simulink model "ssp_ad_scan"  (Simulink 6.5)
settings: Solver=VariableStepDiscrete  SolverMode=SingleTasking  StartTime=0.0  StopTime=10  RelTol=1e-3
undefined symbols (not defined in the file or in its folder): gcbh, xlBlockLoadCallback, xlGetSimulinkPeriod
libraries: xbsIndex_r4 x111, nort_sysgenlib x19
(part 1 of 2)
settings Model: Creator=nort  LastModifiedBy=nort
settings DebuggingCC: MultiTaskDSMMsg=warning  MultiTaskCondExecSysMsg=none
settings RTWCC: IncludeERTFirstTime=on

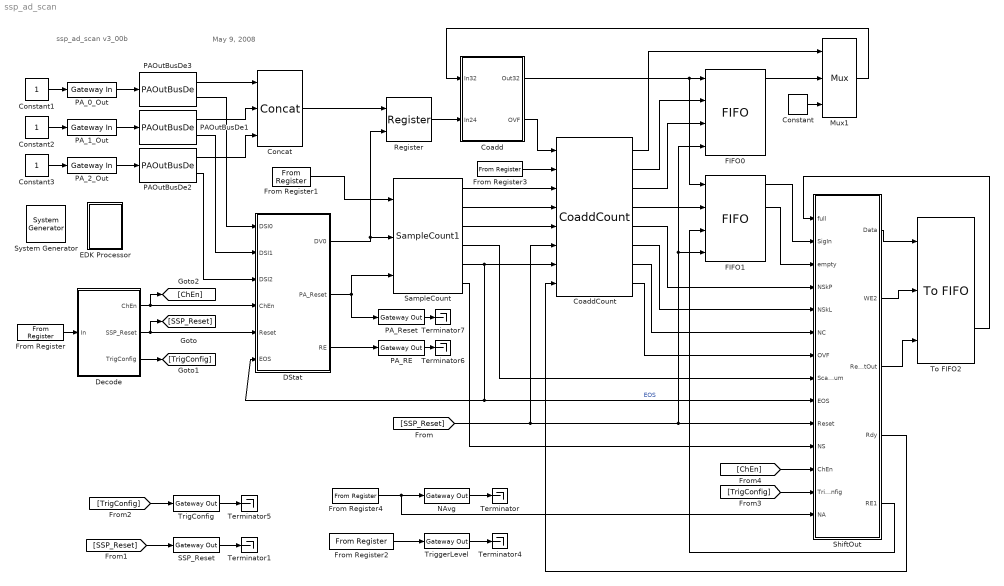
== system ssp_ad_scan ==
  note: May 9, 2008
  note: ssp_ad_scan v3_00b
  " System Generator" : xbsIndex_r4/ System Generator  Tag=genX  SystemSampleTime=-1  xilinxfamily=virtex4  part=xc4vlx25  speed=-10  package=ff668  synthesis_tool=XST  directory=./netlist  testbench=off  simulink_period=1  sysclk_period=10  incr_netlist=off  trim_vbits=Everywhere in SubSystem  dbl_ovrd=According to Block Masks  core_generation=According to Block Masks  run_coregen=off  deprecated_control=off  eval_field=0  block_type=sysgen
      settings: block_version=8.2
  Coadd : Subsystem
  CoaddCount : nort_sysgenlib/CoaddCount  SystemSampleTime=-1
  Concat : xbsIndex_r4/Concat  num_inputs=3  dbl_ovrd=off  block_type=concat
      settings: block_version=9.2.01
  Constant : xbsIndex_r4/Constant  arith_type=Unsigned  const=0  n_bits=96  bin_pt=0  explicit_period=off  period=1  equ=P=C  opselect=C  inp2=PCIN>>17  opr=+  inp1=P  carry=CIN  dbl_ovrd=off  block_type=constant
      settings: block_version=9.2.01
  Constant1 : Constant  Value=1  OutDataType=sfix(16)  ConRadixGroup=Use specified scaling  OutScaling=2^0  SampleTime=inf  FramePeriod=inf
  Constant2 : Constant  Value=1  OutDataType=sfix(16)  ConRadixGroup=Use specified scaling  OutScaling=2^0  SampleTime=inf  FramePeriod=inf
  Constant3 : Constant  Value=1  OutDataType=sfix(16)  ConRadixGroup=Use specified scaling  OutScaling=2^0  SampleTime=inf  FramePeriod=inf
  DStat : Subsystem
  Decode : Subsystem
  EDK Processor : Subsystem  LoadFcn=xlBlockLoadCallback(gcbh);  mask(Xilinx EDK Processor Block){xmp=, proc=, xbd=, mode=EDK pcore generation, MemVisToProc=<qt bgcolor="#FFFFFF"><div><img src="C:\Xilinx91i\dsptools\9.2.01.1028\sysgen\data\images\registerplus.gif"> &lt;&lt;Control&gt;&gt;<br></div><div><img src="C:\Xilinx91i\dsptools\9.2.01.1028\sysgen\data\images\registerminus.gif"> &lt;&lt;NAvg&gt;&gt;<br> <img src="C:\Xilinx91i\dsptools\9.2.01.1028\sysgen\data\images\parameters.gif"> Type : UFix_8_0<br></div><div><img src="C:\Xilinx91i\dsptools\9.2.01.1028\sysgen\data\images\registerplus.gif"> &lt;&lt;NetSamples&gt;&gt;<br></div><div><img src="C:\Xilinx91i\dsptools\9.2.01.1028\sysgen\data\images\registerplus.gif"> &lt;&lt;TriggerLevel&gt;&gt;<br></div><div><img src="C:\Xilinx91i\dsptools\9.2.01.1028\sysgen\data\images\registerplus.gif"> &lt;&lt;NCoadd&gt;&gt;<br></div><div><img src="C:\Xilinx91i\dsptools\9.2.01.1028\sysgen\data\images\fifoplus.gif"> &lt;&lt;SrcSignal&gt;&gt;<br></div></qt>, AvailableMemories=<empty>, launchGDB_sgadvanced=, launchGDB=off, cosim_mode_sgadvanced=, cosim_mode=Single Step, portInterfaceTable={'exposed'=>[],'portdir'=>[],'portname'=>[],'shortname'=>[]}, bus_type_sgadvanced=, bus_type=FSL, baseaddr=0x80000000, baseaddr_lock_sgadvanced=, baseaddr_lock=off, internalPortList={}, resetPolarity=0, memxtable={'mlist'=>['ssp_ad_scan/From Register','ssp_ad_scan/From Register4','ssp_ad_scan/From Register1','ssp_ad_scan/From Register2','ssp_ad_scan/From Register3','ssp_ad_scan/To FIFO2'],'mlname'=>['\'Control\'','\'NAvg\'','\'NetSamples\'','\'TriggerLevel\'','\'NCoadd\'','\'SrcSignal\''],'mlstate'=>[0.00000000000000000,1.0000000000000000,0.00000000000000000,0.00000000000000000,0.00000000000000000,0.00000000000000000]}, procinfo={'xmliface'=>'Xilinx//microblaze//iface.xml'}, fslifaceports=[0,0], memmapdirty=off, blockname=ssp_ad_scan_EDK_Processor, triggeringFunction=main, usermodels=, userCosimTriggers=, has_advanced_control=0, sggui_pos=20,20,383,488, block_type=edkprocessor, block_version=2.2, sg_icon_stat=42,58,-1,-1,white,blue,0,0, sg_mask_display=|, sg_list_contents={'table'=>{'AvailableMemories'=>'popup(<empty>)','userSelections'=>{'AvailableMemories'=>'<empty>'}}}, sg_blockgui_xml=}
      mask sg_mask_display=|
      | fprintf('','COMMENT: begin icon graphics');
      | patch([0 42 42 0 ],[0 0 58 58 ],[0.77 0.82 0.91]);
      | patch([10 3 13 3 10 21 24 27 39 30 21 14 24 14 21 30 39 27 24 21 10 ],[13 20 30 40 47 47 44 47 47 38 47 40 30 20 13 22 13 13 16 13 13 ],[0.98 0.96 0.92]);
      | plot([0 0 42 42 0 ],[0 58 58 0 0 ]);
      | fprintf('','COMMENT: end icon graphics');
      | fprintf('','COMMENT: begin icon text');
      | fprintf('','COMMENT: end icon text');
      mask prompts: xmp "EDK project"; proc "Processor type"; xbd "Target board"; mode "Configure processor for"; MemVisToProc ""; AvailableMemories "Available memories"; launchGDB_sgadvanced ""; launchGDB "Launch GDB"; cosim_mode_sgadvanced ""; cosim_mode "Co-simulation mode"; portInterfaceTable ""; bus_type_sgadvanced ""; bus_type "Bus Type"; baseaddr "Base Address"; baseaddr_lock_sgadvanced ""; baseaddr_lock "lock"; internalPortList ""; resetPolarity ""; memxtable ""; procinfo ""; fslifaceports ""; memmapdirty ""; blockname ""; triggeringFunction ""; usermodels ""; userCosimTriggers ""; has_advanced_control ""; sggui_pos ""; block_type ""; block_version ""; sg_icon_stat ""; sg_mask_display ""; sg_list_contents ""; sg_blockgui_xml ""
      mask help: Xilinx EDK Processor
      mask init:
      | try
      |   tmp_gcb = gcb;
      |   tmp_gcbh = gcbh;
      |   xlMungeMaskParams;
      |   serialized_declarations = '{}';
      |   xledkprocessor_init();
      |   ptable_ = xlblockprep(get_param(tmp_gcb, 'MaskWSVariables'));
      | catch
      |   global dbgsysgen;
      |   if(~isempty(dbgsysgen) && dbgsysgen)
      |     e = regexprep(lasterr, '\n', '\nError: ');
      |     disp(['Error: While running MaskInit code on block ' tmp_gcb ': ' e]);
      |     error(e);
      |   end
      | end
      settings: CopyFcn=xlProcBlockCopyCallback(gcbh);xlBlockMoveCallback(gcbh);  DeleteFcn=xlDestroyGui(gcbh);  ModelCloseFcn=xlDestroyGui(gcbh);  PreSaveFcn=xlBlockPreSaveCallback(gcbh);  PostSaveFcn=xlBlockPostSaveCallback(gcbh);  NameChangeFcn=xlProcBlockCallbacks('namechange',gcbh);  DestroyFcn=xlDestroyGui(gcbh);  OpenFcn=bh=gcbh;xlProcBlockCallbacks('populatesharedmemorylistbox',bh);xlOpenGui(bh, 'edkprocessor_gui.xml', @xlProcBlockEnablement, @xlProcBlockAction)  CloseFcn=xlDestroyGui(gcbh);  MoveFcn=xlBlockMoveCallback(gcbh);
      mask Help: eval('');xlDoc('-book','sysgen','-topic','EDK_Processor');
      mask StyleString: edit,edit,edit,popup(EDK pcore generation|HDL netlisting),edit,popup(<empty>),edit,checkbox,edit,popup(Single Step|Asynchronous),edit,edit,popup(PLB|FSL),edit,edit,checkbox,edit,edit,edit,edit,edit,edit,edit,edit,edit,edit,edit,edit,edit,edit,edit,edit,edit,edit
      mask Display:
      | fprintf('','COMMENT: begin icon graphics');
      | patch([0 42 42 0 ],[0 0 58 58 ],[0.77 0.82 0.91]);
      | patch([10 3 13 3 10 21 24 27 39 30 21 14 24 14 21 30 39 27 24 21 10 ],[13 20 30 40 47 47 44 47 47 38 47 40 30 20 13 22 13 13 16 13 13 ],[0.98 0.96 0.92]);
      | plot([0 0 42 42 0 ],[0 58 58 0 0 ]);
      | fprintf('','COMMENT: end icon graphics');
      | fprintf('','COMMENT: begin icon text');
      | 
      | fprintf('','COMMENT: end icon text');
  FIFO0 : xbsIndex_r4/FIFO  depth=4K  percent_nbits=1  rst=on  en=off  use_dcount=off  use_almost_empty=off  almost_empty_thresh=2  use_almost_full=off  almost_full_thresh=14  dbl_ovrd=off  mem_type=Block RAM  block_type=fifo
      settings: block_version=9.2.01
  FIFO1 : xbsIndex_r4/FIFO  depth=4K  percent_nbits=1  rst=on  en=off  use_dcount=off  use_almost_empty=off  almost_empty_thresh=2  use_almost_full=off  almost_full_thresh=14  dbl_ovrd=off  mem_type=Block RAM  block_type=fifo
      settings: block_version=9.2.01
  From Register : xbsIndex_r4/From Register  shared_memory_name='Control'  init=0  period=1  ownership=Locally owned and initialized  arith_type=Unsigned  n_bits=8  bin_pt=0  dbl_ovrd=off  block_type=fromreg
      settings: AttributesFormatString=<< %<shared_memory_name> >>  infoedit="Register block that reads data to a shared memory register.  Delay of one sample period."  block_version=9.2.01
  From Register1 : xbsIndex_r4/From Register  shared_memory_name='NetSamples'  init=0  period=1  ownership=Locally owned and initialized  arith_type=Unsigned  n_bits=12  bin_pt=0  dbl_ovrd=off  block_type=fromreg
      settings: AttributesFormatString=From Register\n<< %<shared_memory_name> >>  infoedit="Register block that reads data to a shared memory register.  Delay of one sample period."  block_version=8.2
  From Register2 : xbsIndex_r4/From Register  shared_memory_name='TriggerLevel'  init=0  period=1  ownership=Locally owned and initialized  arith_type="Signed  (2's comp)"  n_bits=16  bin_pt=0  dbl_ovrd=off  block_type=fromreg
      settings: AttributesFormatString=From Register\n<< %<shared_memory_name> >>  infoedit="Register block that reads data to a shared memory register.  Delay of one sample period."  block_version=9.1.01
  From Register3 : xbsIndex_r4/From Register  shared_memory_name='NCoadd'  init=0  period=1  ownership=Locally owned and initialized  arith_type=Unsigned  n_bits=14  bin_pt=0  dbl_ovrd=off  block_type=fromreg
      settings: AttributesFormatString=<< %<shared_memory_name> >>  infoedit="Register block that reads data to a shared memory register.  Delay of one sample period."  block_version=9.2.01
  From Register4 : xbsIndex_r4/From Register  shared_memory_name='NAvg'  init=0  period=1  ownership=Locally owned and initialized  arith_type=Unsigned  n_bits=8  bin_pt=0  dbl_ovrd=off  block_type=fromreg
      settings: AttributesFormatString=<< %<shared_memory_name> >>  infoedit="Register block that reads data to a shared memory register.  Delay of one sample period."  block_version=9.2.01
  Mux1 : xbsIndex_r4/Mux  inputs=2  en=off  latency=0  precision=Full  arith_type=Unsigned  n_bits=16  bin_pt=14  quantization=Truncate  overflow=Wrap  dbl_ovrd=off  block_type=mux
      settings: block_version=9.2.01
  NAvg : xbsIndex_r4/Gateway Out  hdl_port=on  timing_constraint=None  locs_specified=off  LOCs={}  block_type=gatewayout
      settings: infoedit="Gateway out block.  Converts Xilinx fixed point inputs into ouputs of type Simulink integer, double, or fixed point.<P><P>Hardware notes:  In hardware these blocks become top level output ports or are discarded, depending on how they are configured."  block_version=9.2.01
  PAOutBusDe1 : nort_sysgenlib/PAOutBusDe  SystemSampleTime=-1
  PAOutBusDe2 : nort_sysgenlib/PAOutBusDe  SystemSampleTime=-1
  PAOutBusDe3 : nort_sysgenlib/PAOutBusDe  SystemSampleTime=-1
  PA_0_Out : xbsIndex_r4/Gateway In  arith_type=Unsigned  n_bits=29  bin_pt=0  quantization="Round  (unbiased: +/- Inf)"  overflow=Wrap  period=1  dbl_ovrd=off  timing_constraint=Data Rate  locs_specified=off  LOCs={}  block_type=gatewayin
      settings: infoedit="Gateway in block.  Converts inputs of type Simulink integer, double and fixed point to  Xilinx fixed point type.<P><P>Hardware notes:  In hardware these blocks become top level input ports."
  PA_1_Out : xbsIndex_r4/Gateway In  arith_type=Unsigned  n_bits=29  bin_pt=0  quantization="Round  (unbiased: +/- Inf)"  overflow=Wrap  period=1  dbl_ovrd=off  timing_constraint=Data Rate  locs_specified=off  LOCs={}  block_type=gatewayin
      settings: infoedit="Gateway in block.  Converts inputs of type Simulink integer, double and fixed point to  Xilinx fixed point type.<P><P>Hardware notes:  In hardware these blocks become top level input ports."
  PA_2_Out : xbsIndex_r4/Gateway In  arith_type=Unsigned  n_bits=29  bin_pt=0  quantization="Round  (unbiased: +/- Inf)"  overflow=Wrap  period=1  dbl_ovrd=off  timing_constraint=Data Rate  locs_specified=off  LOCs={}  block_type=gatewayin
      settings: infoedit="Gateway in block.  Converts inputs of type Simulink integer, double and fixed point to  Xilinx fixed point type.<P><P>Hardware notes:  In hardware these blocks become top level input ports."
  PA_RE : xbsIndex_r4/Gateway Out  hdl_port=on  timing_constraint=None  locs_specified=off  LOCs={}  block_type=gatewayout
      settings: infoedit="Gateway out block.  Converts Xilinx fixed point inputs into ouputs of type Simulink integer, double, or fixed point.<P><P>Hardware notes:  In hardware these blocks become top level output ports or are discarded, depending on how they are configured."  block_version=9.2.01
  PA_Reset : xbsIndex_r4/Gateway Out  hdl_port=on  timing_constraint=None  locs_specified=off  LOCs={}  block_type=gatewayout
      settings: infoedit="Gateway out block.  Converts Xilinx fixed point inputs into ouputs of type Simulink integer, double, or fixed point.<P><P>Hardware notes:  In hardware these blocks become top level output ports or are discarded, depending on how they are configured."  block_version=9.2.01
  Register : xbsIndex_r4/Register  init=0  rst=off  en=on  dbl_ovrd=off  block_type=register
      settings: block_version=9.2.01
  "SSP_Reset\t" : xbsIndex_r4/Gateway Out  hdl_port=on  timing_constraint=None  locs_specified=off  LOCs={}  block_type=gatewayout
      settings: infoedit="Gateway out block.  Converts Xilinx fixed point inputs into ouputs of type Simulink integer, double, or fixed point.<P><P>Hardware notes:  In hardware these blocks become top level output ports or are discarded, depending on how they are configured."  block_version=9.2.01
  SampleCount : nort_sysgenlib/SampleCount1  SystemSampleTime=-1
  ShiftOut : Subsystem
  Terminator{,1,4..7} (6 alike) : Terminator
  To FIFO2 : xbsIndex_r4/To FIFO  shared_memory_name='SrcSignal'  ownership=Locally owned  depth=512  percent_nbits=1  has_arst=on  explicit_data_type=on  arith_type=Unsigned  n_bits=32  bin_pt=0  dbl_ovrd=off  mem_type=Block RAM  block_type=tofifo
      settings: AttributesFormatString=To FIFO\n<< %<shared_memory_name> >>  infoedit=First-in-first-out (FIFO) block that writes FIFO data to shared memory storage.  block_version=8.2
  TrigConfig : xbsIndex_r4/Gateway Out  hdl_port=on  timing_constraint=None  locs_specified=off  LOCs={}  block_type=gatewayout
      settings: infoedit="Gateway out block.  Converts Xilinx fixed point inputs into ouputs of type Simulink integer, double, or fixed point.<P><P>Hardware notes:  In hardware these blocks become top level output ports or are discarded, depending on how they are configured."  block_version=9.2.01
  TriggerLevel : xbsIndex_r4/Gateway Out  hdl_port=on  timing_constraint=None  locs_specified=off  LOCs={}  block_type=gatewayout
      settings: infoedit="Gateway out block.  Converts Xilinx fixed point inputs into ouputs of type Simulink integer, double, or fixed point.<P><P>Hardware notes:  In hardware these blocks become top level output ports or are discarded, depending on how they are configured."  block_version=9.2.01
  wires:
  From Register1/1 -> SampleCount/1
  From Register/1 -> Decode/1(In)
  From Register4/1 -> NAvg/1, ShiftOut/14(NA)
  NAvg/1 -> Terminator/1
  Constant1/1 -> PA_0_Out/1
  From Register2/1 -> TriggerLevel/1
  TriggerLevel/1 -> Terminator4/1
  TrigConfig/1 -> Terminator5/1
  Constant2/1 -> PA_1_Out/1
  Constant3/1 -> PA_2_Out/1
  Decode/1(ChEn) -> [ChEn], DStat/4(ChEn)
  DStat/1(DV0) -> Register/2, SampleCount/2
  Concat/1 -> Register/1
  Coadd/1(Out32) -> FIFO0/1, FIFO1/1
  Register/1 -> Coadd/2(In24)
  Decode/3(TrigConfig) -> [TrigConfig]
  FIFO0/1 -> Mux1/2
  Constant/1 -> Mux1/3
  Mux1/1 -> Coadd/1(In32)
  PA_1_Out/1 -> PAOutBusDe1/1
  PA_2_Out/1 -> PAOutBusDe2/1
  PAOutBusDe1/1 -> Concat/2
  PAOutBusDe2/1 -> Concat/3
  PAOutBusDe1/2 -> DStat/2(DSI1)
  PAOutBusDe2/2 -> DStat/3(DSI2)
  PA_RE/1 -> Terminator6/1
  DStat/3(RE) -> PA_RE/1
  PA_Reset/1 -> Terminator7/1
  DStat/2(PA_Reset) -> PA_Reset/1, SampleCount/3
  Decode/2(SSP_Reset) -> [SSP_Reset], DStat/5(Reset)
  SampleCount/5 -> ShiftOut/9(EOS), DStat/6(EOS), CoaddCount/7  "EOS"
  FIFO1/2 -> ShiftOut/3(empty)
  SampleCount/3 -> CoaddCount/5
  From Register3/1 -> CoaddCount/2
  CoaddCount/1 -> Mux1/1
  SampleCount/2 -> CoaddCount/4
  CoaddCount/2 -> FIFO0/2
  CoaddCount/4 -> FIFO1/2
  FIFO1/1 -> ShiftOut/2(SigIn)
  ShiftOut/2(WE2) -> To FIFO2/2
  ShiftOut/1(Data) -> To FIFO2/1
  To FIFO2/2 -> ShiftOut/1(full)
  CoaddCount/5 -> ShiftOut/4(NSkP)
  CoaddCount/6 -> ShiftOut/5(NSkL)
  CoaddCount/7 -> ShiftOut/6(NC)
  SampleCount/4 -> ShiftOut/8(ScanNum)
  CoaddCount/8 -> ShiftOut/7(OVF)
  Coadd/2(OVF) -> CoaddCount/1
  SampleCount/6 -> ShiftOut/11(NS)
  ShiftOut/5(RE1) -> FIFO1/3
  SampleCount/1 -> CoaddCount/3
  CoaddCount/3 -> FIFO0/3
  ShiftOut/3(ResetOut) -> To FIFO2/3
  PAOutBusDe3/2 -> DStat/1(DSI0)
  PA_0_Out/1 -> PAOutBusDe3/1
  PAOutBusDe3/1 -> Concat/1
  ShiftOut/4(Rdy) -> CoaddCount/8
  [SSP_Reset] -> CoaddCount/6, ShiftOut/10(Reset), FIFO1/4, FIFO0/4
  "SSP_Reset\t"/1 -> Terminator1/1
  [SSP_Reset] -> "SSP_Reset\t"/1
  [TrigConfig] -> TrigConfig/1
  [TrigConfig] -> ShiftOut/13(TrigConfig)
  [ChEn] -> ShiftOut/12(ChEn)

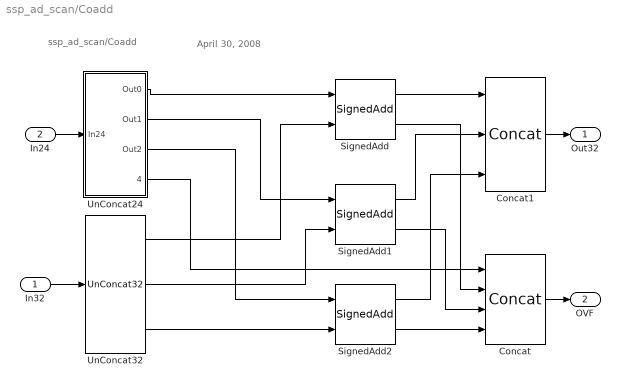
== system ssp_ad_scan/Coadd ==
  note: ssp_ad_scan/Coadd
  note: April 30, 2008
  In32 : Inport
  In24 : Inport  Port=2
  Concat : xbsIndex_r4/Concat  num_inputs=4  dbl_ovrd=off  block_type=concat
      settings: block_version=9.2.01
  Concat1 : xbsIndex_r4/Concat  num_inputs=3  dbl_ovrd=off  block_type=concat
      settings: block_version=9.2.01
  SignedAdd : nort_sysgenlib/SignedAdd  SystemSampleTime=-1
  SignedAdd1 : nort_sysgenlib/SignedAdd  SystemSampleTime=-1
  SignedAdd2 : nort_sysgenlib/SignedAdd  SystemSampleTime=-1
  UnConcat24 : Subsystem
  UnConcat32 : nort_sysgenlib/UnConcat32  SystemSampleTime=-1
  Out32 : Outport
  OVF : Outport  Port=2
  wires:
  SignedAdd2/1 -> Concat1/3
  SignedAdd1/1 -> Concat1/2
  SignedAdd/1 -> Concat1/1
  UnConcat24/3(Out2) -> SignedAdd2/1
  UnConcat24/2(Out1) -> SignedAdd1/1
  UnConcat24/1(Out0) -> SignedAdd/1
  UnConcat32/1 -> SignedAdd/2
  Concat1/1 -> Out32/1
  UnConcat32/2 -> SignedAdd1/2
  UnConcat32/3 -> SignedAdd2/2
  In32/1 -> UnConcat32/1
  In24/1 -> UnConcat24/1(In24)
  Concat/1 -> OVF/1
  SignedAdd/2 -> Concat/2
  SignedAdd1/2 -> Concat/3
  SignedAdd2/2 -> Concat/4
  UnConcat24/4(PAOVF) -> Concat/1

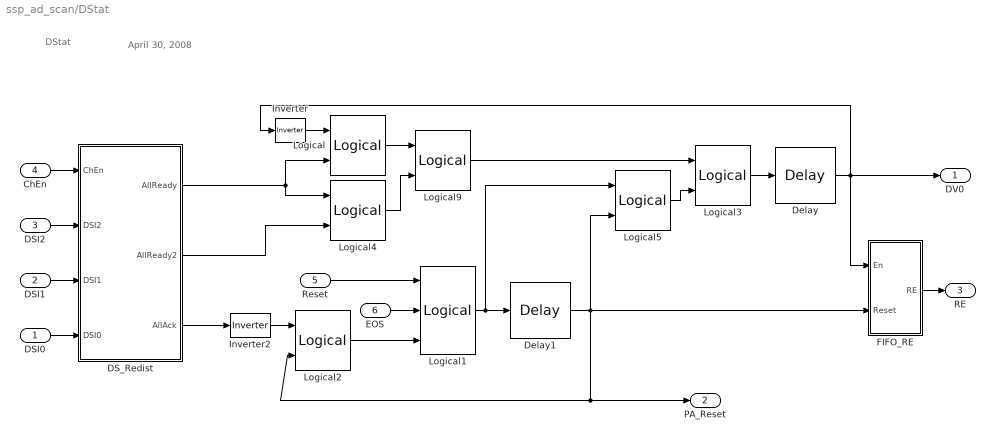
== system ssp_ad_scan/DStat ==
  note: DStat
  note: April 30, 2008
  DSI0 : Inport
  DSI1 : Inport  Port=2
  DSI2 : Inport  Port=3
  ChEn : Inport  Port=4
  Reset : Inport  Port=5
  EOS : Inport  Port=6
  DS_Redist : Subsystem
  Delay : xbsIndex_r4/Delay  en=off  latency=1  dbl_ovrd=off  reg_retiming=off  block_type=delay
      settings: block_version=9.2.01
  Delay1 : xbsIndex_r4/Delay  en=off  latency=1  dbl_ovrd=off  reg_retiming=off  block_type=delay
      settings: block_version=9.2.01
  FIFO_RE : Subsystem
  Inverter : xbsIndex_r4/Inverter  en=off  latency=0  dbl_ovrd=off  block_type=inv
      settings: block_version=9.2.01
  Inverter2 : xbsIndex_r4/Inverter  en=off  latency=0  dbl_ovrd=off  block_type=inv
      settings: block_version=9.2.01
  Logical : xbsIndex_r4/Logical  logical_function=AND  inputs=2  en=off  latency=0  precision=Full  arith_type=Unsigned  n_bits=16  bin_pt=0  align_bp=on  dbl_ovrd=off  block_type=logical
      settings: block_version=9.2.01
  Logical1 : xbsIndex_r4/Logical  logical_function=OR  inputs=3  en=off  latency=0  precision=Full  arith_type=Unsigned  n_bits=16  bin_pt=0  align_bp=on  dbl_ovrd=off  block_type=logical
      settings: block_version=9.2.01
  Logical2 : xbsIndex_r4/Logical  logical_function=AND  inputs=2  en=off  latency=0  precision=Full  arith_type=Unsigned  n_bits=16  bin_pt=0  align_bp=on  dbl_ovrd=off  block_type=logical
      settings: block_version=9.2.01
  Logical3 : xbsIndex_r4/Logical  logical_function=NOR  inputs=2  en=off  latency=0  precision=Full  arith_type=Unsigned  n_bits=16  bin_pt=0  align_bp=on  dbl_ovrd=off  block_type=logical
      settings: block_version=9.2.01
  Logical4 : xbsIndex_r4/Logical  logical_function=AND  inputs=2  en=off  latency=0  precision=Full  arith_type=Unsigned  n_bits=16  bin_pt=0  align_bp=on  dbl_ovrd=off  block_type=logical
      settings: block_version=9.2.01
  Logical5 : xbsIndex_r4/Logical  logical_function=OR  inputs=2  en=off  latency=0  precision=Full  arith_type=Unsigned  n_bits=16  bin_pt=0  align_bp=on  dbl_ovrd=off  block_type=logical
      settings: block_version=9.2.01
  Logical9 : xbsIndex_r4/Logical  logical_function=NOR  inputs=2  en=off  latency=0  precision=Full  arith_type=Unsigned  n_bits=16  bin_pt=0  align_bp=on  dbl_ovrd=off  block_type=logical
      settings: block_version=9.2.01
  DV0 : Outport
  PA_Reset : Outport  Port=2
  RE : Outport  Port=3
  wires:
  DS_Redist/1(AllReady) -> Logical4/1, Logical/2
  Delay/1 -> DV0/1, Inverter/1, FIFO_RE/1(En)
  FIFO_RE/1(RE) -> RE/1
  DSI0/1 -> DS_Redist/4(DSI0)
  Inverter/1 -> Logical/1
  Logical/1 -> Logical9/1
  Logical9/1 -> Logical3/1
  DSI1/1 -> DS_Redist/3(DSI1)
  DSI2/1 -> DS_Redist/2(DSI2)
  Reset/1 -> Logical1/1
  DS_Redist/3(AllAck) -> Inverter2/1
  Logical1/1 -> Delay1/1, Logical5/1
  Inverter2/1 -> Logical2/1
  Delay1/1 -> Logical5/2, PA_Reset/1, Logical2/2, FIFO_RE/2(Reset)
  EOS/1 -> Logical1/2
  Logical3/1 -> Delay/1
  ChEn/1 -> DS_Redist/1(ChEn)
  Logical4/1 -> Logical9/2
  DS_Redist/2(AllReady2) -> Logical4/2
  Logical5/1 -> Logical3/2
  Logical2/1 -> Logical1/3

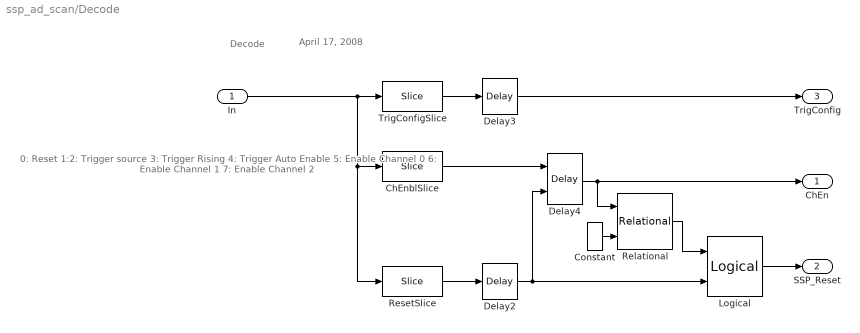
== system ssp_ad_scan/Decode ==
  note: Decode
  note: 0: Reset
      | 1:2: Trigger source
      | 3: Trigger Rising
      | 4: Trigger Auto Enable
      | 5: Enable Channel 0
      | 6: Enable Channel 1
      | 7: Enable Channel 2
  note: April 17, 2008
  In : Inport
  ChEnblSlice : xbsIndex_r4/Slice  nbits=3  boolean_output=off  mode=Lower Bit Location + Width  bit1=0  base1=MSB of Input  bit0=5  base0=LSB of Input  dbl_ovrd=off  block_type=slice
      settings: infoedit="Extracts a given range of bits from each input sample and presents it at the output.  The output type is ordinarily unsigned with binary point at zero, but can be Boolean when the slice is one bit wide.<P><P>Hardware notes: In hardware this block costs nothing."  block_version=8.2
  Constant : xbsIndex_r4/Constant  arith_type=Unsigned  const=0  n_bits=3  bin_pt=0  explicit_period=off  period=1  equ=P=C  opselect=C  inp2=PCIN>>17  opr=+  inp1=P  carry=CIN  dbl_ovrd=off  block_type=constant
      settings: block_version=9.2.01
  Delay2 : xbsIndex_r4/Delay  en=off  latency=1  dbl_ovrd=off  reg_retiming=off  block_type=delay
      settings: block_version=9.1.01
  Delay3 : xbsIndex_r4/Delay  en=off  latency=1  dbl_ovrd=off  reg_retiming=off  block_type=delay
      settings: block_version=9.1.01
  Delay4 : xbsIndex_r4/Delay  en=on  latency=1  dbl_ovrd=off  reg_retiming=off  block_type=delay
      settings: block_version=9.1.01
  Logical : xbsIndex_r4/Logical  logical_function=OR  inputs=2  en=off  latency=0  precision=Full  arith_type=Unsigned  n_bits=16  bin_pt=0  align_bp=on  dbl_ovrd=off  block_type=logical
      settings: block_version=9.2.01
  Relational : xbsIndex_r4/Relational  mode=a=b  en=off  latency=0  dbl_ovrd=off  block_type=relational
      settings: block_version=9.2.01
  ResetSlice : xbsIndex_r4/Slice  nbits=1  boolean_output=on  mode=Lower Bit Location + Width  bit1=0  base1=MSB of Input  bit0=0  base0=LSB of Input  dbl_ovrd=off  block_type=slice
      settings: infoedit="Extracts a given range of bits from each input sample and presents it at the output.  The output type is ordinarily unsigned with binary point at zero, but can be Boolean when the slice is one bit wide.<P><P>Hardware notes: In hardware this block costs nothing."  block_version=8.2
  TrigConfigSlice : xbsIndex_r4/Slice  nbits=4  boolean_output=off  mode=Lower Bit Location + Width  bit1=0  base1=MSB of Input  bit0=1  base0=LSB of Input  dbl_ovrd=off  block_type=slice
      settings: infoedit="Extracts a given range of bits from each input sample and presents it at the output.  The output type is ordinarily unsigned with binary point at zero, but can be Boolean when the slice is one bit wide.<P><P>Hardware notes: In hardware this block costs nothing."  block_version=8.2
  ChEn : Outport
  SSP_Reset : Outport  Port=2
  TrigConfig : Outport  Port=3
  wires:
  In/1 -> TrigConfigSlice/1, ChEnblSlice/1, ResetSlice/1
  ResetSlice/1 -> Delay2/1
  TrigConfigSlice/1 -> Delay3/1
  Delay2/1 -> Delay4/2, Logical/2
  Delay3/1 -> TrigConfig/1
  ChEnblSlice/1 -> Delay4/1
  Delay4/1 -> ChEn/1, Relational/1
  Constant/1 -> Relational/2
  Relational/1 -> Logical/1
  Logical/1 -> SSP_Reset/1

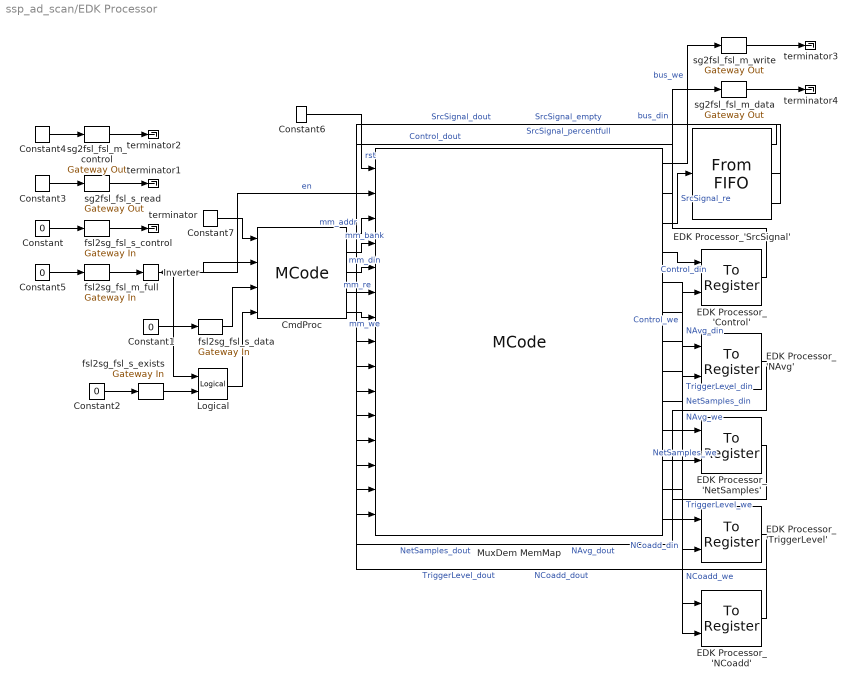
== system ssp_ad_scan/EDK Processor ==
  CmdProc : xbsIndex_r4/MCode  mfname=xlCmdProc  explicit_period=off  period=1  dbl_ovrd=off  enable_stdout=off  enable_debug=off  suppress_output=1  defparams={'gBankTop',27,'gBankBot',20 ,'gAddrTop',19,'gAddrBot',0,'gValTop',21,'gValBot',0,'gRegTop',27,'gRegBot',20,'gOpTop',30,'gOpBot',28}  hide_port_list={}  block_type=mcode
      settings: block_version=9.2.01
  Constant{,1..2,5} (4 alike) : Constant  Value=0  OutDataType=sfix(16)  ConRadixGroup=Use specified scaling  OutScaling=2^0  SampleTime=inf  FramePeriod=inf
  Constant3 : xbsIndex_r4/Constant  arith_type=Unsigned  const=1  n_bits=1  bin_pt=0  explicit_period=off  period=xlGetSimulinkPeriod(gcb)  equ=P=C  opselect=C  inp2=PCIN>>17  opr=+  inp1=P  carry=CIN  dbl_ovrd=off  block_type=constant
      settings: block_version=9.2.01
  Constant4 : xbsIndex_r4/Constant  arith_type=Unsigned  const=0  n_bits=1  bin_pt=0  explicit_period=off  period=xlGetSimulinkPeriod(gcb)  equ=P=C  opselect=C  inp2=PCIN>>17  opr=+  inp1=P  carry=CIN  dbl_ovrd=off  block_type=constant
      settings: block_version=9.2.01
  Constant6 : xbsIndex_r4/Constant  arith_type=Boolean  const=0  n_bits=1  bin_pt=0  explicit_period=on  period=xlGetSimulinkPeriod(gcb)  equ=P=C  opselect=C  inp2=PCIN>>17  opr=+  inp1=P  carry=CIN  dbl_ovrd=off  block_type=constant
      settings: block_version=9.2.01
  Constant7 : xbsIndex_r4/Constant  arith_type=Boolean  const=0  n_bits=1  bin_pt=0  explicit_period=on  period=xlGetSimulinkPeriod(gcb)  equ=P=C  opselect=C  inp2=PCIN>>17  opr=+  inp1=P  carry=CIN  dbl_ovrd=off  block_type=constant
      settings: block_version=9.2.01
  EDK Processor_'Control' : xbsIndex_r4/To Register  shared_memory_name='Control'  init=0  ownership=Owned and initialized elsewhere  explicit_data_type=on  arith_type=Unsigned  n_bits=8  bin_pt=0  dbl_ovrd=off  block_type=toreg
      settings: AttributesFormatString=<< %<shared_memory_name> >>  infoedit="Register block that writes data to a shared memory register.  Delay of one sample period."  block_version=9.2.01
  EDK Processor_'NAvg' : xbsIndex_r4/To Register  shared_memory_name='NAvg'  init=0  ownership=Owned and initialized elsewhere  explicit_data_type=on  arith_type=Unsigned  n_bits=8  bin_pt=0  dbl_ovrd=off  block_type=toreg
      settings: AttributesFormatString=<< %<shared_memory_name> >>  infoedit="Register block that writes data to a shared memory register.  Delay of one sample period."  block_version=9.2.01
  EDK Processor_'NCoadd' : xbsIndex_r4/To Register  shared_memory_name='NCoadd'  init=0  ownership=Owned and initialized elsewhere  explicit_data_type=on  arith_type=Unsigned  n_bits=14  bin_pt=0  dbl_ovrd=off  block_type=toreg
      settings: AttributesFormatString=<< %<shared_memory_name> >>  infoedit="Register block that writes data to a shared memory register.  Delay of one sample period."  block_version=9.2.01
  EDK Processor_'NetSamples' : xbsIndex_r4/To Register  shared_memory_name='NetSamples'  init=0  ownership=Owned and initialized elsewhere  explicit_data_type=on  arith_type=Unsigned  n_bits=12  bin_pt=0  dbl_ovrd=off  block_type=toreg
      settings: AttributesFormatString=<< %<shared_memory_name> >>  infoedit="Register block that writes data to a shared memory register.  Delay of one sample period."  block_version=9.2.01
  EDK Processor_'SrcSignal' : xbsIndex_r4/From FIFO  shared_memory_name='SrcSignal'  ownership=Owned elsewhere  depth=512  percent_nbits=9  has_arst=off  arith_type=Unsigned  n_bits=32  bin_pt=0  dbl_ovrd=off  mem_type=Block RAM  block_type=fromfifo
      settings: AttributesFormatString=<< %<shared_memory_name> >>  infoedit=First-in-first-out (FIFO) block that reads FIFO data from shared memory storage.  block_version=9.2.01
  EDK Processor_'TriggerLevel' : xbsIndex_r4/To Register  shared_memory_name='TriggerLevel'  init=0  ownership=Owned and initialized elsewhere  explicit_data_type=on  arith_type="Signed  (2's comp)"  n_bits=16  bin_pt=0  dbl_ovrd=off  block_type=toreg
      settings: AttributesFormatString=<< %<shared_memory_name> >>  infoedit="Register block that writes data to a shared memory register.  Delay of one sample period."  block_version=9.2.01
  Inverter : xbsIndex_r4/Inverter  en=off  latency=0  dbl_ovrd=off  block_type=inv
      settings: block_version=9.2.01
  Logical : xbsIndex_r4/Logical  logical_function=AND  inputs=2  en=off  latency=0  precision=Full  arith_type=Unsigned  n_bits=16  bin_pt=0  align_bp=on  dbl_ovrd=off  block_type=logical
      settings: block_version=9.2.01
  MuxDem MemMap : xbsIndex_r4/MCode  mfname=ssp_ad_scan_EDK_Processor_MemMap  explicit_period=off  period=1  dbl_ovrd=off  enable_stdout=off  enable_debug=off  suppress_output=1  defparams={}  hide_port_list={}  block_type=mcode
      settings: block_version=9.2.01
  fsl2sg_fsl_m_full : xbsIndex_r4/Gateway In  arith_type=Unsigned  n_bits=1  bin_pt=0  quantization="Round  (unbiased: +/- Inf)"  overflow=Saturate  period=xlGetSimulinkPeriod(gcb)  dbl_ovrd=off  timing_constraint=None  locs_specified=off  LOCs={}  block_type=gatewayin
      settings: infoedit="Gateway in block.  Converts inputs of type Simulink integer, double and fixed point to  Xilinx fixed point type.<P><P>Hardware notes:  In hardware these blocks become top level input ports."  block_version=9.2.01
  fsl2sg_fsl_s_control : xbsIndex_r4/Gateway In  arith_type=Unsigned  n_bits=1  bin_pt=0  quantization="Round  (unbiased: +/- Inf)"  overflow=Saturate  period=xlGetSimulinkPeriod(gcb)  dbl_ovrd=off  timing_constraint=None  locs_specified=off  LOCs={}  block_type=gatewayin
      settings: infoedit="Gateway in block.  Converts inputs of type Simulink integer, double and fixed point to  Xilinx fixed point type.<P><P>Hardware notes:  In hardware these blocks become top level input ports."  block_version=9.2.01
  fsl2sg_fsl_s_data : xbsIndex_r4/Gateway In  arith_type=Unsigned  n_bits=32  bin_pt=0  quantization="Round  (unbiased: +/- Inf)"  overflow=Saturate  period=xlGetSimulinkPeriod(gcb)  dbl_ovrd=off  timing_constraint=None  locs_specified=off  LOCs={}  block_type=gatewayin
      settings: infoedit="Gateway in block.  Converts inputs of type Simulink integer, double and fixed point to  Xilinx fixed point type.<P><P>Hardware notes:  In hardware these blocks become top level input ports."  block_version=9.2.01
  fsl2sg_fsl_s_exists : xbsIndex_r4/Gateway In  arith_type=Unsigned  n_bits=1  bin_pt=0  quantization="Round  (unbiased: +/- Inf)"  overflow=Saturate  period=xlGetSimulinkPeriod(gcb)  dbl_ovrd=off  timing_constraint=None  locs_specified=off  LOCs={}  block_type=gatewayin
      settings: infoedit="Gateway in block.  Converts inputs of type Simulink integer, double and fixed point to  Xilinx fixed point type.<P><P>Hardware notes:  In hardware these blocks become top level input ports."  block_version=9.2.01
  sg2fsl_fsl_m_control : xbsIndex_r4/Gateway Out  hdl_port=on  timing_constraint=None  locs_specified=off  LOCs={}  block_type=gatewayout
      settings: infoedit="Gateway out block.  Converts Xilinx fixed point inputs into ouputs of type Simulink integer, double, or fixed point.<P><P>Hardware notes:  In hardware these blocks become top level output ports or are discarded, depending on how they are configured."  block_version=9.2.01
  sg2fsl_fsl_m_data : xbsIndex_r4/Gateway Out  hdl_port=on  timing_constraint=None  locs_specified=off  LOCs={}  block_type=gatewayout
      settings: infoedit="Gateway out block.  Converts Xilinx fixed point inputs into ouputs of type Simulink integer, double, or fixed point.<P><P>Hardware notes:  In hardware these blocks become top level output ports or are discarded, depending on how they are configured."  block_version=9.2.01
  sg2fsl_fsl_m_write : xbsIndex_r4/Gateway Out  hdl_port=on  timing_constraint=None  locs_specified=off  LOCs={}  block_type=gatewayout
      settings: infoedit="Gateway out block.  Converts Xilinx fixed point inputs into ouputs of type Simulink integer, double, or fixed point.<P><P>Hardware notes:  In hardware these blocks become top level output ports or are discarded, depending on how they are configured."  block_version=9.2.01
  sg2fsl_fsl_s_read : xbsIndex_r4/Gateway Out  hdl_port=on  timing_constraint=None  locs_specified=off  LOCs={}  block_type=gatewayout
      settings: infoedit="Gateway out block.  Converts Xilinx fixed point inputs into ouputs of type Simulink integer, double, or fixed point.<P><P>Hardware notes:  In hardware these blocks become top level output ports or are discarded, depending on how they are configured."  block_version=9.2.01
  terminator{,1..4} (5 alike) : Terminator
  wires:
  Inverter/1 -> CmdProc/2, Logical/1, MuxDem MemMap/2  "en"
  CmdProc/5 -> MuxDem MemMap/7  "mm_we"
  CmdProc/4 -> MuxDem MemMap/6  "mm_re"
  CmdProc/3 -> MuxDem MemMap/5  "mm_din"
  CmdProc/2 -> MuxDem MemMap/4  "mm_bank"
  CmdProc/1 -> MuxDem MemMap/3  "mm_addr"
  Logical/1 -> CmdProc/4
  fsl2sg_fsl_s_data/1 -> CmdProc/3
  Constant7/1 -> CmdProc/1
  Constant6/1 -> MuxDem MemMap/1  "rst"
  fsl2sg_fsl_s_exists/1 -> Logical/2
  fsl2sg_fsl_m_full/1 -> Inverter/1
  Constant5/1 -> fsl2sg_fsl_m_full/1
  sg2fsl_fsl_m_data/1 -> terminator4/1
  MuxDem MemMap/2 -> sg2fsl_fsl_m_data/1  "bus_din"
  sg2fsl_fsl_m_write/1 -> terminator3/1
  MuxDem MemMap/1 -> sg2fsl_fsl_m_write/1  "bus_we"
  sg2fsl_fsl_m_control/1 -> terminator2/1
  Constant4/1 -> sg2fsl_fsl_m_control/1
  sg2fsl_fsl_s_read/1 -> terminator1/1
  Constant3/1 -> sg2fsl_fsl_s_read/1
  Constant2/1 -> fsl2sg_fsl_s_exists/1
  Constant1/1 -> fsl2sg_fsl_s_data/1
  fsl2sg_fsl_s_control/1 -> terminator/1
  Constant/1 -> fsl2sg_fsl_s_control/1
  EDK Processor_'SrcSignal'/3 -> MuxDem MemMap/9  "SrcSignal_empty"
  EDK Processor_'SrcSignal'/2 -> MuxDem MemMap/8  "SrcSignal_percentfull"
  EDK Processor_'SrcSignal'/1 -> MuxDem MemMap/15  "SrcSignal_dout"
  MuxDem MemMap/3 -> EDK Processor_'SrcSignal'/1  "SrcSignal_re"
  EDK Processor_'NCoadd'/1 -> MuxDem MemMap/14  "NCoadd_dout"
  MuxDem MemMap/13 -> EDK Processor_'NCoadd'/2  "NCoadd_we"
  MuxDem MemMap/8 -> EDK Processor_'NCoadd'/1  "NCoadd_din"
  EDK Processor_'TriggerLevel'/1 -> MuxDem MemMap/13  "TriggerLevel_dout"
  MuxDem MemMap/12 -> EDK Processor_'TriggerLevel'/2  "TriggerLevel_we"
  MuxDem MemMap/7 -> EDK Processor_'TriggerLevel'/1  "TriggerLevel_din"
  EDK Processor_'NetSamples'/1 -> MuxDem MemMap/12  "NetSamples_dout"
  MuxDem MemMap/11 -> EDK Processor_'NetSamples'/2  "NetSamples_we"
  MuxDem MemMap/6 -> EDK Processor_'NetSamples'/1  "NetSamples_din"
  EDK Processor_'NAvg'/1 -> MuxDem MemMap/11  "NAvg_dout"
  MuxDem MemMap/10 -> EDK Processor_'NAvg'/2  "NAvg_we"
  MuxDem MemMap/5 -> EDK Processor_'NAvg'/1  "NAvg_din"
  EDK Processor_'Control'/1 -> MuxDem MemMap/10  "Control_dout"
  MuxDem MemMap/9 -> EDK Processor_'Control'/2  "Control_we"
  MuxDem MemMap/4 -> EDK Processor_'Control'/1  "Control_din"

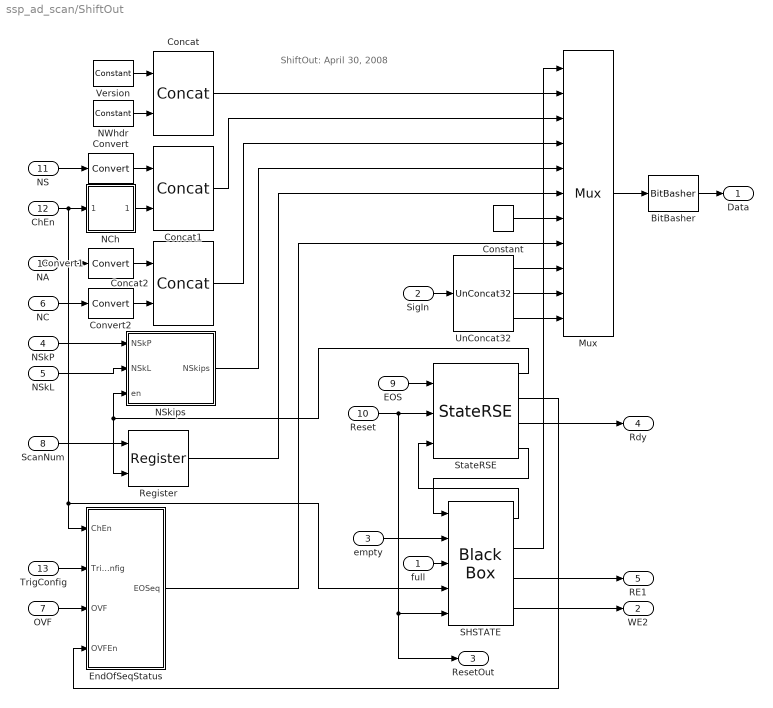
== system ssp_ad_scan/ShiftOut ==
  note: ShiftOut: April 30, 2008
  full : Inport
  SigIn : Inport  Port=2
  empty : Inport  Port=3
  NSkP : Inport  Port=4
  NSkL : Inport  Port=5
  NC : Inport  Port=6
  OVF : Inport  Port=7
  ScanNum : Inport  Port=8
  EOS : Inport  Port=9
  Reset : Inport  Port=10
  NS : Inport  Port=11
  ChEn : Inport  Port=12
  TrigConfig : Inport  Port=13
  NA : Inport  Port=14
  BitBasher : xbsIndex_r4/BitBasher  bitexpr=|  display_expr=off  sr_1=1  arith_type1=Unsigned  bin_pt1=0  sr_2=2  arith_type2=Unsigned  bin_pt2=0  sr_3=3  arith_type3=Unsigned  bin_pt3=0  sr_4=4  arith_type4=Unsigned  bin_pt4=0  dbl_ovrd=off  block_type=bitbasher
      | <html><head><meta name="qrichtext" content="1" /></head><body style="font-size:8pt;font-family:MS Shell Dlg">
      | <p>BE={LE[7:0],LE[15:8],LE[23:16],LE[31:24]}</p>
      | </body></html>
      settings: block_version=8.2
      settings: infoedit=|
      | Allows
      |      extraction, concatenation and augmentation of bits
  Concat : xbsIndex_r4/Concat  num_inputs=2  dbl_ovrd=off  block_type=concat
      settings: block_version=9.2.01
  Concat1 : xbsIndex_r4/Concat  num_inputs=2  dbl_ovrd=off  block_type=concat
      settings: block_version=9.2.01
  Concat2 : xbsIndex_r4/Concat  num_inputs=2  dbl_ovrd=off  block_type=concat
      settings: block_version=9.2.01
  Constant : xbsIndex_r4/Constant  arith_type=Unsigned  const=0  n_bits=32  bin_pt=0  explicit_period=off  period=1  equ=P=C  opselect=C  inp2=PCIN>>17  opr=+  inp1=P  carry=CIN  dbl_ovrd=off  block_type=constant
      settings: block_version=9.2.01
  Convert : xbsIndex_r4/Convert  arith_type=Unsigned  n_bits=16  bin_pt=0  quantization=Truncate  overflow=Wrap  latency=0  dbl_ovrd=off  pipeline=off  block_type=convert
      settings: block_version=9.2.01
  Convert1 : xbsIndex_r4/Convert  arith_type=Unsigned  n_bits=16  bin_pt=0  quantization=Truncate  overflow=Wrap  latency=0  dbl_ovrd=off  pipeline=off  block_type=convert
      settings: block_version=9.2.01
  Convert2 : xbsIndex_r4/Convert  arith_type=Unsigned  n_bits=16  bin_pt=0  quantization=Truncate  overflow=Wrap  latency=0  dbl_ovrd=off  pipeline=off  block_type=convert
      settings: block_version=9.2.01
  EndOfSeqStatus : Subsystem
  Mux : xbsIndex_r4/Mux  inputs=10  en=off  latency=0  precision=User Defined  arith_type="Signed  (2's comp)"  n_bits=32  bin_pt=0  quantization=Truncate  overflow=Saturate  dbl_ovrd=off  block_type=mux
      settings: block_version=8.2
  NCh : Subsystem
  NSkips : Subsystem
  NWhdr : xbsIndex_r4/Constant  arith_type=Unsigned  const=6  n_bits=16  bin_pt=0  explicit_period=off  period=1  equ=P=C  opselect=C  inp2=PCIN>>17  opr=+  inp1=P  carry=CIN  dbl_ovrd=off  block_type=constant
      settings: block_version=9.2.01
  Register : xbsIndex_r4/Register  init=0  rst=off  en=on  dbl_ovrd=off  block_type=register
      settings: block_version=9.2.01
  SHSTATE : xbsIndex_r4/Black Box  init_code=SHSTATE_config  sim_method=Inactive  block_type=blackbox2
      settings: infoedit="Incorporates black box HDL and simulation model into a System Generator design.<P><P>You must supply a Black Box with certain information about the HDL component you would like to bring into System Generator. This information is provided through a Matlab function.<P><P>When \"Simulation mode\" is set to \"Inactive\", you will typically want to provide a separate simulation model by using a Simulation Multiplexer.<P>When \"Simulation mode\" is set to \"External co-simulator\", you must include a ModelSim block in the design."  block_version=9.2.01
  StateRSE : nort_sysgenlib/StateRSE  SystemSampleTime=-1
  UnConcat32 : nort_sysgenlib/UnConcat32  SystemSampleTime=-1
  Version : xbsIndex_r4/Constant  arith_type=Unsigned  const=0  n_bits=16  bin_pt=0  explicit_period=off  period=1  equ=P=C  opselect=C  inp2=PCIN>>17  opr=+  inp1=P  carry=CIN  dbl_ovrd=off  block_type=constant
      settings: block_version=9.2.01
  Data : Outport
  WE2 : Outport  Port=2
  ResetOut : Outport  Port=3
  Rdy : Outport  Port=4
  RE1 : Outport  Port=5
  wires:
  Mux/1 -> BitBasher/1
  BitBasher/1 -> Data/1
  Reset/1 -> ResetOut/1, SHSTATE/5, StateRSE/2
  Version/1 -> Concat/1
  NWhdr/1 -> Concat/2
  Concat/1 -> Mux/2
  NS/1 -> Convert/1
  Convert/1 -> Concat1/1
  ChEn/1 -> NCh/1(ChEn), EndOfSeqStatus/1(ChEn), SHSTATE/4
  NCh/1(NCh) -> Concat1/2
  Concat1/1 -> Mux/3
  NA/1 -> Convert1/1
  NC/1 -> Convert2/1
  Concat2/1 -> Mux/4
  Convert1/1 -> Concat2/1
  Convert2/1 -> Concat2/2
  NSkips/1(NSkips) -> Mux/5
  NSkP/1 -> NSkips/1(NSkP)
  NSkL/1 -> NSkips/2(NSkL)
  ScanNum/1 -> Register/1
  Register/1 -> Mux/6
  Constant/1 -> Mux/7
  OVF/1 -> EndOfSeqStatus/3(OVF)
  TrigConfig/1 -> EndOfSeqStatus/2(TrigConfig)
  EndOfSeqStatus/1(EOSeq) -> Mux/8
  UnConcat32/1 -> Mux/9
  UnConcat32/2 -> Mux/10
  UnConcat32/3 -> Mux/11
  SigIn/1 -> UnConcat32/1
  StateRSE/4 -> SHSTATE/1
  EOS/1 -> StateRSE/1
  empty/1 -> SHSTATE/2
  full/1 -> SHSTATE/3
  StateRSE/2 -> EndOfSeqStatus/4(OVFEn)
  StateRSE/1 -> Register/2, NSkips/3(en)
  SHSTATE/4 -> WE2/1
  SHSTATE/3 -> RE1/1
  SHSTATE/2 -> Mux/1
  SHSTATE/1 -> StateRSE/3
  StateRSE/3 -> Rdy/1

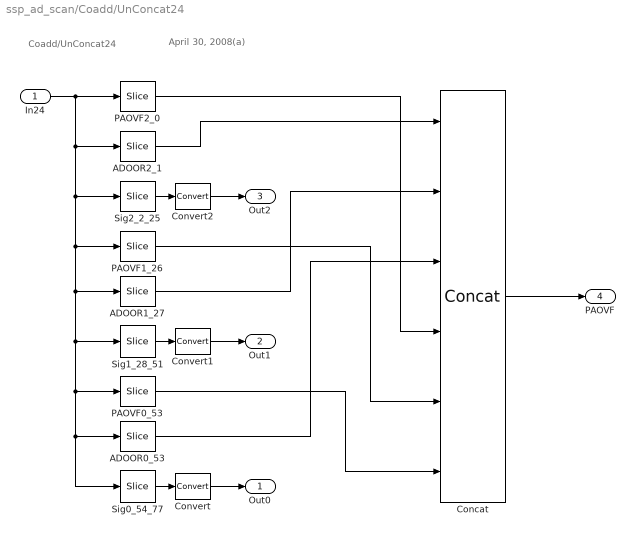
== system ssp_ad_scan/Coadd/UnConcat24 ==
  note: Coadd/UnConcat24
  note: April 30, 2008(a)
  In24 : Inport
  ADOOR0_53 : xbsIndex_r4/Slice  nbits=1  boolean_output=off  mode=Lower Bit Location + Width  bit1=0  base1=MSB of Input  bit0=53  base0=LSB of Input  dbl_ovrd=off  block_type=slice
      settings: infoedit="Extracts a given range of bits from each input sample and presents it at the output.  The output type is ordinarily unsigned with binary point at zero, but can be Boolean when the slice is one bit wide.<P><P>Hardware notes: In hardware this block costs nothing."  block_version=9.2.01
  ADOOR1_27 : xbsIndex_r4/Slice  nbits=1  boolean_output=off  mode=Lower Bit Location + Width  bit1=0  base1=MSB of Input  bit0=27  base0=LSB of Input  dbl_ovrd=off  block_type=slice
      settings: infoedit="Extracts a given range of bits from each input sample and presents it at the output.  The output type is ordinarily unsigned with binary point at zero, but can be Boolean when the slice is one bit wide.<P><P>Hardware notes: In hardware this block costs nothing."  block_version=9.2.01
  ADOOR2_1 : xbsIndex_r4/Slice  nbits=1  boolean_output=off  mode=Lower Bit Location + Width  bit1=0  base1=MSB of Input  bit0=1  base0=LSB of Input  dbl_ovrd=off  block_type=slice
      settings: infoedit="Extracts a given range of bits from each input sample and presents it at the output.  The output type is ordinarily unsigned with binary point at zero, but can be Boolean when the slice is one bit wide.<P><P>Hardware notes: In hardware this block costs nothing."  block_version=9.2.01
  Concat : xbsIndex_r4/Concat  num_inputs=6  dbl_ovrd=off  block_type=concat
      settings: block_version=9.2.01
  Convert : xbsIndex_r4/Convert  arith_type="Signed  (2's comp)"  n_bits=24  bin_pt=0  quantization=Truncate  overflow=Wrap  latency=0  dbl_ovrd=off  pipeline=off  block_type=convert
      settings: block_version=9.2.01
  Convert1 : xbsIndex_r4/Convert  arith_type="Signed  (2's comp)"  n_bits=24  bin_pt=0  quantization=Truncate  overflow=Wrap  latency=0  dbl_ovrd=off  pipeline=off  block_type=convert
      settings: block_version=9.2.01
  Convert2 : xbsIndex_r4/Convert  arith_type="Signed  (2's comp)"  n_bits=24  bin_pt=0  quantization=Truncate  overflow=Wrap  latency=0  dbl_ovrd=off  pipeline=off  block_type=convert
      settings: block_version=9.2.01
  PAOVF0_53 : xbsIndex_r4/Slice  nbits=1  boolean_output=off  mode=Lower Bit Location + Width  bit1=0  base1=MSB of Input  bit0=52  base0=LSB of Input  dbl_ovrd=off  block_type=slice
      settings: infoedit="Extracts a given range of bits from each input sample and presents it at the output.  The output type is ordinarily unsigned with binary point at zero, but can be Boolean when the slice is one bit wide.<P><P>Hardware notes: In hardware this block costs nothing."  block_version=9.2.01
  PAOVF1_26 : xbsIndex_r4/Slice  nbits=1  boolean_output=off  mode=Lower Bit Location + Width  bit1=0  base1=MSB of Input  bit0=0  base0=LSB of Input  dbl_ovrd=off  block_type=slice
      settings: infoedit="Extracts a given range of bits from each input sample and presents it at the output.  The output type is ordinarily unsigned with binary point at zero, but can be Boolean when the slice is one bit wide.<P><P>Hardware notes: In hardware this block costs nothing."  block_version=9.2.01
  PAOVF2_0 : xbsIndex_r4/Slice  nbits=1  boolean_output=off  mode=Lower Bit Location + Width  bit1=0  base1=MSB of Input  bit0=0  base0=LSB of Input  dbl_ovrd=off  block_type=slice
      settings: infoedit="Extracts a given range of bits from each input sample and presents it at the output.  The output type is ordinarily unsigned with binary point at zero, but can be Boolean when the slice is one bit wide.<P><P>Hardware notes: In hardware this block costs nothing."  block_version=9.2.01
  Sig0_54_77 : xbsIndex_r4/Slice  nbits=24  boolean_output=off  mode=Lower Bit Location + Width  bit1=0  base1=MSB of Input  bit0=54  base0=LSB of Input  dbl_ovrd=off  block_type=slice
      settings: infoedit="Extracts a given range of bits from each input sample and presents it at the output.  The output type is ordinarily unsigned with binary point at zero, but can be Boolean when the slice is one bit wide.<P><P>Hardware notes: In hardware this block costs nothing."  block_version=9.2.01
  Sig1_28_51 : xbsIndex_r4/Slice  nbits=24  boolean_output=off  mode=Lower Bit Location + Width  bit1=0  base1=MSB of Input  bit0=28  base0=LSB of Input  dbl_ovrd=off  block_type=slice
      settings: infoedit="Extracts a given range of bits from each input sample and presents it at the output.  The output type is ordinarily unsigned with binary point at zero, but can be Boolean when the slice is one bit wide.<P><P>Hardware notes: In hardware this block costs nothing."  block_version=9.2.01
  Sig2_2_25 : xbsIndex_r4/Slice  nbits=24  boolean_output=off  mode=Lower Bit Location + Width  bit1=0  base1=MSB of Input  bit0=2  base0=LSB of Input  dbl_ovrd=off  block_type=slice
      settings: infoedit="Extracts a given range of bits from each input sample and presents it at the output.  The output type is ordinarily unsigned with binary point at zero, but can be Boolean when the slice is one bit wide.<P><P>Hardware notes: In hardware this block costs nothing."  block_version=9.2.01
  Out0 : Outport
  Out1 : Outport  Port=2
  Out2 : Outport  Port=3
  PAOVF : Outport  Port=4
  wires:
  Sig0_54_77/1 -> Convert/1
  Sig1_28_51/1 -> Convert1/1
  Sig2_2_25/1 -> Convert2/1
  Convert/1 -> Out0/1
  Convert1/1 -> Out1/1
  Convert2/1 -> Out2/1
  In24/1 -> PAOVF2_0/1, Sig0_54_77/1, ADOOR0_53/1, PAOVF0_53/1, Sig1_28_51/1, ADOOR1_27/1, PAOVF1_26/1, Sig2_2_25/1, ADOOR2_1/1
  Concat/1 -> PAOVF/1
  ADOOR2_1/1 -> Concat/1
  ADOOR1_27/1 -> Concat/2
  ADOOR0_53/1 -> Concat/3
  PAOVF2_0/1 -> Concat/4
  PAOVF1_26/1 -> Concat/5
  PAOVF0_53/1 -> Concat/6

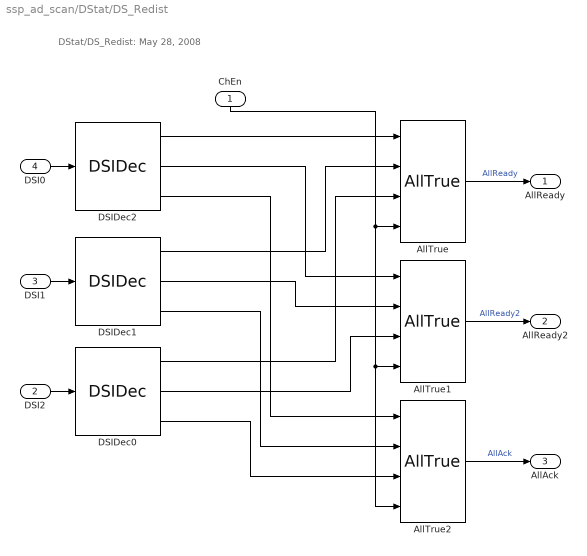
== system ssp_ad_scan/DStat/DS_Redist ==
  note: DStat/DS_Redist: May 28, 2008
  ChEn : Inport  Orientation=down
  DSI2 : Inport  Port=2
  DSI1 : Inport  Port=3
  DSI0 : Inport  Port=4
  AllTrue : nort_sysgenlib/AllTrue  SystemSampleTime=-1
  AllTrue1 : nort_sysgenlib/AllTrue  SystemSampleTime=-1
  AllTrue2 : nort_sysgenlib/AllTrue  SystemSampleTime=-1
  DSIDec0 : nort_sysgenlib/DSIDec  SystemSampleTime=-1
  DSIDec1 : nort_sysgenlib/DSIDec  SystemSampleTime=-1
  DSIDec2 : nort_sysgenlib/DSIDec  SystemSampleTime=-1
  AllReady : Outport
  AllReady2 : Outport  Port=2
  AllAck : Outport  Port=3
  wires:
  DSIDec2/1 -> AllTrue/1
  DSIDec1/1 -> AllTrue/2
  DSIDec0/1 -> AllTrue/3
  DSIDec2/2 -> AllTrue1/1
  ChEn/1 -> AllTrue/4, AllTrue1/4, AllTrue2/4
  DSIDec1/2 -> AllTrue1/2
  DSIDec0/2 -> AllTrue1/3
  DSIDec2/3 -> AllTrue2/1
  DSIDec1/3 -> AllTrue2/2
  DSIDec0/3 -> AllTrue2/3
  DSI2/1 -> DSIDec0/1
  AllTrue/1 -> AllReady/1  "AllReady"
  DSI1/1 -> DSIDec1/1
  AllTrue1/1 -> AllReady2/1  "AllReady2"
  DSI0/1 -> DSIDec2/1
  AllTrue2/1 -> AllAck/1  "AllAck"

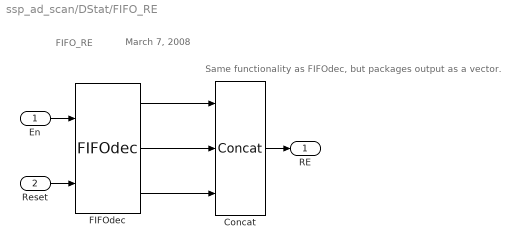
== system ssp_ad_scan/DStat/FIFO_RE ==
  note: FIFO_RE
  note: March 7, 2008
  note: Same functionality as
      | FIFOdec, but packages
      | output as a vector.
  En : Inport
  Reset : Inport  Port=2
  Concat : xbsIndex_r4/Concat  num_inputs=3  dbl_ovrd=off  block_type=concat
      settings: block_version=9.2.01
  FIFOdec : nort_sysgenlib/FIFOdec  SystemSampleTime=-1
  RE : Outport
  wires:
  FIFOdec/1 -> Concat/1
  FIFOdec/2 -> Concat/2
  FIFOdec/3 -> Concat/3
  En/1 -> FIFOdec/1
  Concat/1 -> RE/1
  Reset/1 -> FIFOdec/2
